simulink model "DR18E_Testpult"  (R2017a)
settings: Solver=ode1  StartTime=0.0  StopTime=Inf  FixedStep=0.001  RelTol=1e-3
PostLoadFcn:
  | , if any(exist('dsrtsu_mdlpostloadfcn', 'file') == [2, 3, 6]), try dsrtsu_mdlpostloadfcn('Execute', bdroot); catch fprintf('Error in PostLoadFcn (dsrtsu_mdlpostloadfcn) for model "%s":\n %s\n', bdroot, lasterr); end, end,
model workspace: external: MAT-File C:\Users\DeltaRacing\Documents\dSPACE\MABX_DR18E\Model\DR18E_MABX_Parameter.mat (data not in the file)
values from neighbouring files (symbols this model uses):
  am = 1/Ts    (= 1)    [DR18E_MABX_Parameter.m]
  bm = K/Ts    (= 0.05)    [DR18E_MABX_Parameter.m]
  cf = 41350    [DR18E_MABX_Parameter.m]
  cr = 41350    [DR18E_MABX_Parameter.m]
  Derating_HV_Battery_Kapa = 1    [DR18E_MABX_Parameter.m]
  Derating_Start_km = 16    [DR18E_MABX_Parameter.m]
  Drive_Mode = 0    [DR18E_MABX_Parameter.m]
  g = 1    [DR18E_MABX_Parameter.m]
  Gas_Modus = 2    [DR18E_MABX_Parameter.m]
  HV_Power_max = 80    [DR18E_MABX_Parameter.m]
  i_Getriebe = 3.3    [DR18E_MABX_Parameter.m]
  i_Lenkgetriebe = 4.32    [DR18E_MABX_Parameter.m]
  K_SET = 1    [DR18E_MABX_Parameter.m]
  Kapazitaet_HV_Battery_kWh = 6.6    [DR18E_MABX_Parameter.m]
  KW_T_Soll = 37    [DR18E_MABX_Parameter.m]
  lf = 1.2    [DR18E_MABX_Parameter.m]
  lr = 1.15    [DR18E_MABX_Parameter.m]
  m = mdriver + mvehicle    (= 310)    [DR18E_MABX_Parameter.m]
  M_max = 150    [DR18E_MABX_Parameter.m]
  Power_Limit_onoff = 0    [DR18E_MABX_Parameter.m]
  Reifenradius = 0.2351    [DR18E_MABX_Parameter.m]
  Strecke_Endu_km = 22    [DR18E_MABX_Parameter.m]
  TC_Decr_Gas = 0.00005    (= 5e-05)    [DR18E_MABX_Parameter.m]
  TC_Derivative = 0.4    [DR18E_MABX_Parameter.m]
  TC_Incr_Gas = 0.005    [DR18E_MABX_Parameter.m]
  TC_On = 0    [DR18E_MABX_Parameter.m]
  TC_Relay_Off = 0.065    [DR18E_MABX_Parameter.m]
  TC_Relay_On = 0.07    [DR18E_MABX_Parameter.m]
  TV_Mode = 2    [DR18E_MABX_Parameter.m]
  TV_On = 0    [DR18E_MABX_Parameter.m]
  TV_Override = 1    [DR18E_MABX_Parameter.m]
  y = 0.8    [DR18E_MABX_Parameter.m]
undefined symbols (not defined in the file or in its folder): D, DiscIntNeverNeededParam, I, K_OL, P
libraries: simulink x288, rtican x100, rtiusbflightreclib x40, rti1401lib_dio_type3 x10, simulink_extras x10, rti1401lib_adc_type4 x8, rti1401lib_II_base x7
(part 2 of 27)

== system DR18E_Testpult/Verarbeitung ==
  note: Einheit checken
  note: ist das hier der richtige Relaisstatus
  note: Aufpassen, es gibt eine GLV-Gesamtspannung
      | bzw. Zellspannungen
  main : Inport
  Alarme : Subsystem
  BMS_Monitor : Subsystem
  Bremse : Subsystem
  Bus Creator : BusCreator  Inputs=25
  Bus Creator1 : BusCreator  Inputs=7
  Bus Selector : BusSelector  OutputSignals=RX_SensorboardFront.RX_Bremse,RX_SensorboardFront.RX_Gas
  Bus Selector3 : BusSelector  OutputSignals=BMS_State.HV_Voltage_total,RX_SensorboardFront.HVCurrent
  Bus Selector6 : BusSelector  OutputSignals=RX_SensorboardMitte.Drehzahlen vorne.RPM_Left,RX_SensorboardMitte.Drehzahlen vorne.RPM_Right,Umrichter.U1.Drehzahl_1min,Umrichter.U2.Drehzahl_1min
  Bus Selector7 : BusSelector  OutputSignals=RX_CANIO.IMD_State,BMS_State.AMS_RelayState,RX_GLVAMS.GLV_Voltage_ges
  Bus Selector8 : BusSelector  OutputSignals=O_coolingEnable
  Bus Selector9 : BusSelector  OutputSignals=RX_SensorboardRear.Water_Temperature_Pump,RX_SensorboardRear.Water_Temperature_Cooler,Umrichter.U1.InverterTemp,Umrichter.U2.InverterTemp,Umrichter.U1.Mot_Temp,Umrichter.U2.Mot_Temp,BMS.STK1-5_Temp,BMS.STK6-10_Temp
  DIS : Subsystem
  DR18E Torque Control : Subsystem
  GLV-Undervoltage : Subsystem
  Gaspedal Check : Subsystem
  MABX RAM : Subsystem
  Precalculations : Subsystem
  SafetyShutdown : Subsystem
  Strom/SOC : Subsystem
  Temperaturregelung1 : Subsystem  SystemSampleTime=0.2
  Umrichter Init Config : Subsystem
  Vehicle State Machine : Subsystem
  Out1 : Outport
  wires:
  Bus Selector9/2 -> Temperaturregelung1/1(Temp Kühlwasser)  "<Water_Temperature_Cooler>"
  Bus Selector3/2 -> Strom/SOC/2(HV_Current)  "<HVCurrent>"
  Bus Selector3/1 -> Strom/SOC/1(HV_Voltage)  "<HV_Voltage_total>"
  [Inputs] -> Alarme/1(In1)
  Bus Selector9/4 -> Temperaturregelung1/3(Temp IGBT Umrichter2)  "<InverterTemp>"
  Bus Selector8/1 -> [O_coolingEnable]  "<O_coolingEnable>"
  [Inputs] -> Bus Selector7/1
  [Inputs] -> Bus Selector3/1
  Bus Selector6/3 -> Precalculations/3(Drehzahl RL)  "<Drehzahl_1min>"
  [Inputs] -> Gaspedal Check/1(Gaspedal)
  [Inputs] -> Bus Selector9/1
  [O_coolingEnable] -> Temperaturregelung1/8(O_coolingEnable)
  Bus Selector6/4 -> Precalculations/4(Drehzahl RR)  "<Drehzahl_1min>"
  Bus Selector9/3 -> Temperaturregelung1/2(Temp IGBT Umrichter1)  "<InverterTemp>"
  SafetyShutdown/1(TorqueRequestLROut) -> Bus Creator/1  "Torque_L_R_Nm"
  Bus Selector6/1 -> Precalculations/1(Drehzahl FL)  "<RPM_Left>"
  [Inputs] -> Precalculations/5("Inputs Bus "), Bus Selector6/1
  Vehicle State Machine/1(Outputs) -> Bus Creator/9, Bus Selector8/1
  Bus Selector9/5 -> Temperaturregelung1/4(Temp Motor 1)  "<Mot_Temp>"
  [Inputs] -> Bus Creator/7, Vehicle State Machine/1(In1)  "Bus_Input"
  Bus Selector9/6 -> Temperaturregelung1/5(Temp Motor 2)  "<Mot_Temp>"
  Bus Selector6/2 -> Precalculations/2(Drehzahl FR)  "<RPM_Right>"
  [Inputs] -> GLV-Undervoltage/1(GLV-Spannung)
  Bus Selector7/3 -> Bus Creator/25  "<GLV_Voltage_ges>"
  Bus Selector7/2 -> Bus Creator/24  "<AMS_RelayState>"
  Bus Creator/1 -> Out1/1
  main/1 -> [Inputs]
  Temperaturregelung1/1(LüfterPWM) -> Bus Creator/17  "LüfterPWM"
  Temperaturregelung1/2(PumpePWM) -> Bus Creator/19  "PumpePWM"
  GLV-Undervoltage/1(GLV-Undervoltage) -> Bus Creator/22
  Bus Selector7/1 -> Bus Creator/23  "<IMD_State>"
  Alarme/1(ErrorCode) -> Bus Creator/14  "ErrorNo"
  [Inputs] -> Bus Selector/1
  Bus Selector/1 -> Bremse/1(Bremse)  "<RX_Bremse>"
  Bus Selector/2 -> Bremse/2(Gaspedal %)  "<RX_Gas>"
  [Bremse_bin] -> Bus Creator/13  "Bremse_bin"
  Alarme/2(Out1) -> Bus Creator/15  "Sicherheitskreis"
  Gaspedal Check/1(Gas_0-1) -> DR18E Torque Control/1(Gas_0-1)
  Precalculations/1(v_kmh) -> Bus Creator1/1  "v_kmh"
  Precalculations/2(Long_Slip_Left) -> Bus Creator1/2  "long_slip_left"
  Precalculations/3(Long_Slip_Right) -> Bus Creator1/3  "long_slip_right"
  Precalculations/4(Outputs Bus) -> Bus Creator1/4  "Bus"
  Bus Creator1/1 -> DIS/1(In1), DR18E Torque Control/2(Inputs)
  Strom/SOC/1(HV_Power_Watt) -> Bus Creator1/5
  DR18E Torque Control/1(MotorTorque Nm) -> SafetyShutdown/1(TorqueRequestLR)
  Temperaturregelung1/3(Lüfter HV Battery) -> Bus Creator/20  "Lüfter HV Battery"
  Bus Selector9/7 -> Temperaturregelung1/6(HV Battery Temp STK 1-5)  "<STK1-5_Temp>"
  Bus Selector9/8 -> Temperaturregelung1/7(HV Battery Temp STK 6-10)  "<STK6-10_Temp>"
  DR18E Torque Control/2(M_max/Motor) -> Bus Creator/3  "M_max"
  MABX RAM/1(TagesmeterMABX_m) -> Bus Creator1/6
  MABX RAM/2(TagesenergieMABX_Wh) -> Bus Creator1/7
  DIS/1(Out1) -> Bus Creator/6  "LED Bar Vektor"
  [Inputs] -> BMS_Monitor/1(In1)

== system DR18E_Testpult/Ausgabe/AMS ==
  Lüfter HV Battery : Inport
  Data Type Conversion4 : DataTypeConversion  OutMin=0  OutMax=1  OutDataTypeStr=double
  Detect Change1 : simulink/Logic and Bit Operations/Detect Change  vinit=0  InputProcessing=Inherited  OutDataTypeStr=boolean
  Gain : Gain  Gain=255
  SIG_FAN_HVBATTERY : rtican/RTICAN Transmit (TX)   Reserved1=[]  Reserved2=[]  Reserved3=[]  Reserved4=[]  SfcnMessage=[]  Msg_Struct=[]  BoardTypeNo=[]  BoardNo=[]  ChannelNo=[]  Parameters=[]  DialogFcn=[]  UnitName=[]  Revision=[]  UnitValues=[]  DSProperties=struct('RTI',struct('Version',uint32(5),'BlockType',struct('isSLSource',uint8(1),'isSLSink',uint8(1),'isHWSource',uint8(0),'isHWSink',uint8(0),'isSetup',uint8(0),'isInline',uint8(1),'isNonInline',uint8(0),'isInterrupt',uint8(0),'isChannelwise',uint8(0)),'IOBoardType','RTICAN','UnitType','MESSAGE','Identifier','TX','DialogType','MSVC','BlockSet','RTICAN','SlaveProcessor','CAN'))  RTIBlockInterface=struct('InputPortsWidth',int32(1),'InputPortsActive',1,'InputPortsName',{{'SIG_FAN_HVBATTERY'}},'InputPortsDataType',{{'SS_DOUBLE'}},'OutputPortsWidth',int32([1 1 1]),'OutputPortsActive',[1 1 1],'OutputPortsName',{{['TX status'],['TX time'],['TX delta time']}},'DialogFcn','rtican_message_interface_gui','BlockDisplay',{{'','center'}},'IconTransparency','on','InitLevel',3,'BlockName',struct('Token',{{'SIG_FAN_HVBATTERY'}}),'SampleTime',{{0.05}},'TriggerPort',{{'none'}},'EnablePort',{{'yes'}})  RTIBlockParameters=struct('BoardTypeNo',{{1,'OFF',[]}},'BoardNo',{{2,'ON',[1 16]}},'ChannelNo',{{1,'ON',[1 2]}},'Parameters',{{struct('DataFileSupport',struct('DataFileSelectedMaster',1,'DataFileSelectedLocal',1,'DataFileName','c:\users\deltaracing\documents\canoe\dr18e\dbc\dr18e.dbc|','DataFileDate',['16-Feb-2019 13:23:09'],'SelectedFile','..\..\..\canoe\dr18e_test\dr18e\dbc\dr18e.dbc','InterfaceFcn','rtican_dbc_file_parser'),'Options',struct('StatusSelected',1,'TimeSelected',1,'DeltaTimeSelected',1,'DelayTimeSelected',0,'DelayTimeTXCommandSelected',0,'EncodeSetUnusedBitsToOne',0,'EnableMsgLoopback',0,'TriggerPort',struct('Selected',0,'TriggerType',2),'EnablePortSelected',1,'SignalOnPortnameSelected',1,'UserCoding',struct('Selected',0,'InterfaceFile','UserEncodingFile','FcnName','UserEncodeFcn','InportSelected',0,'InportWidth',1,'OutportSelected',0,'OutportWidth',1),'TerminationMsg',struct('Selected',0,'Byte0_7','0'),'InitialMsg',struct('Selected',0,'Byte0_7','0')),'Message',struct('MsgOnBlocknameSelected',1,'MsgName','SIG_FAN_HVBATTERY','MsgIdFormat',0,'MsgId',822,'MsgLength',1,'NumSignals',1,'SampleTime',0.05,'StartTime',struct('Selected',0,'Value',0),'AutoRepeatTime',struct('Selected',0,'Value',0.1),'Timeout',struct('Selected',0,'Value',0.1),'DelayTime',struct('Selected',0,'Value',0.1),'Signal',struct('SgnName','SIG_FAN_HVBATTERY','SgnStartBit',0,'SgnLength',8,'ByteLayout',0,'Factor',1,'Offset',0,'SgnComment','','SgnUnit','','Min',0,'Max',255,'SgnType',0,'SLDataType','SS_DOUBLE','DataType',0,'ModeValue',-1),'MsgIdNumFormat',0,'MsgComment',{{''}}),'Version',1.2,'general',struct('isFromLib',0)),'OFF',[]}},'GroupId',{{struct('Group',{{'RTICAN'}},'No',1,'Behavior',{{'NAMECHANGE'}},'BlockType',{{'SINK'}},'NameChangeFlag',0),'OFF',[]}},'SFcnRTICANMessage',{{struct('MsgType','TX','SFcnPortType','Scalar','MsgName','SIG_FAN_HVBATTERY','MsgIdFormat','STD','MsgId',822,'MsgLength',1,'NumSignals',1,'SampleTime',0.05,'StartTime',struct('Selected','no','Value',0),'AutoRepeatTime',struct('Selected','no','Value',0.1),'Timeout',struct('Selected','no','Value',0.1),'Signal',struct('SgnName','SIG_FAN_HVBATTERY','SgnStartBit',0,'SgnLength',8,'ByteLayout',['little endian'],'Factor',1,'Offset',0,'SgnType','standard','SLDataType','SS_DOUBLE','DataType',['unsigned int'],'ModeValue',-1),'StatusSelected','yes','TimeSelected','yes','DeltaTimeSelected','yes','DelayTimeSelected','no','DelayTimeTXCommandSelected','no','EncodeSetUnusedBitsToOne','no','EnableMsgLoopback','no','TriggerPort',struct('Selected','no','TriggerType',2),'EnablePortSelected','yes','UserCoding',struct('Selected','no','InterfaceFile','UserEncodingFile','FcnName','UserEncodeFcn','InportSelected','no','InportWidth',1,'OutportSelected','no','OutportWidth',1),'TerminationMsg',struct('Selected','no','Byte0','0x00','Byte1','0x00','Byte2','0x00','Byte3','0x00','Byte4','0x00','Byte5','0x00','Byte6','0x00','Byte7','0x00'),'InitialMsg',struct('Selected','no','Byte0','0x00','Byte1','0x00','Byte2','0x00','Byte3','0x00','Byte4','0x00','Byte5','0x00','Byte6','0x00','Byte7','0x00'),'BoardType','DS1','BoardNo',2,'ControllerNo',1),'OFF',[]}},'TLCFileName',{{'rtican_tx_message','OFF',[]}})  RTISFcnParameters=struct('SFcnRTICANMessage','struct','TLCFileName','char')  RTIBlockParaDefault=struct('BoardTypeNo',4302,'BoardNo',1,'ChannelNo',1,'Parameters',struct('DataFileSupport',struct('DataFileSelectedMaster',0,'DataFileSelectedLocal',0,'DataFileName','','DataFileDate','','SelectedFile',['<no file selected>']),'Options',struct('StatusSelected',1,'TimeSelected',1,'DeltaTimeSelected',1,'DelayTimeSelected',1,'DelayTimeTXCommandSelected',0,'EncodeSetUnusedBitsToOne',0,'EnableMsgLoopback',0,'TriggerPort',struct('Selected',0,'TriggerType','rising'),'EnablePortSelected',0,'SignalOnPortnameSelected',1,'UserCoding',struct('Selected',0,'InterfaceFile','UserEncodingFile','FcnName','UserEncodeFcn','InportSelected',0,'InportWidth',1,'OutportSelected',0,'OutportWidth',1),'TerminationMsg',struct('Selected',0,'Byte0_7','0'),'InitialMsg',struct('Selected',0,'Byte0_7','0')),'Message',struct('MsgOnBlocknameSelected',0,'MsgName',['TX Message'],'MsgIdFormat',0,'MsgId',100,'MsgLength',8,'NumSignals',1,'SampleTime',-1,'StartTime',struct('Selected',0,'Value',0),'AutoRepeatTime',struct('Selected',0,'Value',0.1),'Timeout',struct('Selected',0,'Value',0.1),'DelayTime',struct('Selected',0,'Value',0.1),'Signal',struct('SgnName',['TX signal'],'SgnStartBit',0,'SgnLength',8,'SgnType',0,'ModeValue',-1,'DataType',0,'SLDataType','SS_DOUBLE','ByteLayout',0,'Factor',1,'Offset',0,'Min',0,'Max',255,'SgnComment',{{}},'SgnUnit',''),'MsgIdNumFormat',0,'MsgComment',{{''}}),'Version',1.2,'general',struct('isFromLib',1)),'GroupId',struct('Group',{{'RTICAN'}},'No',1,'Behavior',{{'NAMECHANGE'}},'BlockType',{{'SINK'}},'NameChangeFlag',0),'SFcnRTICANMessage',struct('MsgType','TX','MsgName',['TX Message'],'MsgIdFormat','STD','MsgId',100,'MsgLength',2,'NumSignals',1,'SampleTime',-1,'StartTime',struct('Selected','no','Value',0),'AutoRepeatTime',struct('Selected','no','Value',0.1),'Timeout',struct('Selected','no','Value',0.1),'DelayTime',struct('Selected','no','Value',0.1),'Signal',struct('SgnName',['TX signal'],'SgnStartBit',0,'SgnLength',8,'SgnType','standard','ModeValue',-1,'DataType',['unsigned int'],'ByteLayout',['little endian'],'SLDataType','SS_DOUBLE','Factor',1,'Offset',0),'StatusSelected','yes','TimeSelected','yes','DeltaTimeSelected','yes','DelayTimeSelected','yes','EnablePortSelected','no','EnableMsgLoopback','no','DelayTimeTXCommandSelected','no','EncodeSetUnusedBitsToOne','no','UserCoding',struct('Selected','no','InterfaceFile','UserDecodingFile','FcnName','UserDecodeFcn','InportSelected','no','InportWidth',1,'OutportSelected','no','OutportWidth',1),'TerminationMsg',struct('Selected','no','Byte0','0x00','Byte1','0x00','Byte2','0x00','Byte3','0x00','Byte4','0x00','Byte5','0x00','Byte6','0x00','Byte7','0x00'),'InitialMsg',struct('Selected','no','Byte0','0x00','Byte1','0x00','Byte2','0x00','Byte3','0x00','Byte4','0x00','Byte5','0x00','Byte6','0x00','Byte7','0x00'),'TriggerPort',struct('Selected','no','TriggerType','rising'),'BoardType','DS4302','BoardNo',1,'ControllerNo',1,'SFcnPortType','Scalar'),'TLCFileName','rtican_tx_message')
      settings: AttributesFormatString=Group Id: RTICAN1\n  SourceProductName=dSPACE RTI CAN Blockset
  Terminator_3 : Terminator
  Transmit OK Detection3 : Subsystem
  wires:
  Transmit OK Detection3/1(TX Warn) -> Terminator_3/1
  SIG_FAN_HVBATTERY/3 -> Transmit OK Detection3/2(TX delta time)
  SIG_FAN_HVBATTERY/1 -> Transmit OK Detection3/1(TX status)
  Lüfter HV Battery/1 -> Data Type Conversion4/1
  Data Type Conversion4/1 -> Gain/1, Detect Change1/1
  Detect Change1/1 -> SIG_FAN_HVBATTERY/Enable
  Gain/1 -> SIG_FAN_HVBATTERY/1
